simulink model "task_4_1"  (R2024a)
settings: Solver=VariableStepAuto  StartTime=0.0  StopTime=20.0  RelTol=1e-3
libraries: simulink x1
settings Model: Creator=alexe  LastModifiedBy=alexe

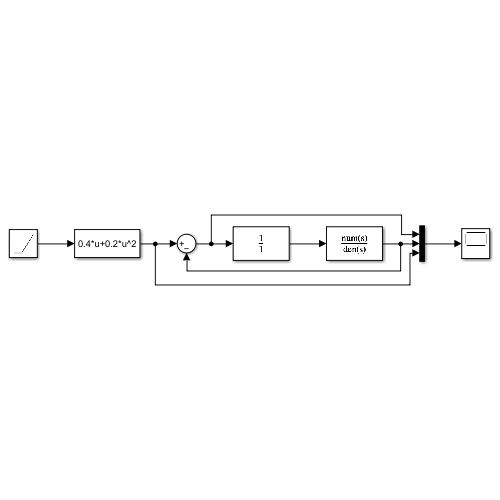
[thumbnail: Simulink's stored preview of the top-level diagram]
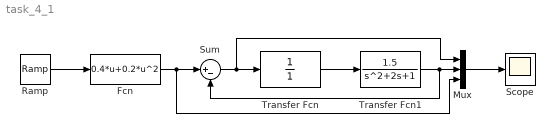
== system task_4_1 ==
  Fcn : Fcn  Expr=0.4*u+0.2*u^2
  Mux : Mux  Inputs=3
  Ramp : simulink/Sources/Ramp  slope=1  start=0  InitialOutput=0
  Scope : Scope
  Sum : Sum  Inputs=|+-
  Transfer Fcn : TransferFcn  Denominator=[1]
  Transfer Fcn1 : TransferFcn  Numerator=[1.5]
  wires:
  Ramp/1 -> Fcn/1
  Fcn/1 -> Mux/3, Sum/1
  Sum/1 -> Mux/1, Transfer Fcn/1
  Transfer Fcn/1 -> Transfer Fcn1/1
  Mux/1 -> Scope/1
  Transfer Fcn1/1 -> Sum/2, Mux/2
